simulink model "QPSK_ad9361_LNA"  (R2017b)
settings: Solver=ode23  StartTime=0.0  StopTime=inf  RelTol=1e-3  EnableMultiTasking=on
PreLoadFcn:
  | addpath('./filterwizard');
  | adi9361_preload(bdroot,'rx');
  | sdrqpsktx = sdrzqpsktxFMC234_init;
  | sdrqpskrx = sdrzqpskrxFMC234_init;
InitFcn:
  | sdrqpsktx = sdrzqpsktxFMC234_init;
  | sdrqpskrx = sdrzqpskrxFMC234_init;
undefined symbols (not defined in the file or in its folder): D, dBval, DCLeak_Matrix, dfilt, fuzz_val, GainImb_Matrix, gcbh, IP2_Matrix, IP3_Matrix, magnitude, rcfiltgaincompat
libraries: simrfV2elements x12, simulink x7, dsparch4 x6, dspmlti4 x5, simrfV2util1 x4, fl_lib x4, simrfV2junction1 x3, dspsrcs4 x3, dspmathops x3, commdigbbndpm3 x3, dspstat3 x3, dspobslib x3
(part 1 of 3)
settings Model: SimulationMode=accelerator  Creator=The MathWorks Inc.  LastModifiedBy=ppradhan
settings DataIOCC: ExternalInput=txWaveform  SaveFormat=StructureWithTime  SaveOutput=off  SignalLogging=off  DSMLogging=off  SaveTime=off  OutputSaveName=rx
settings OptimizationCC: DefaultParameterBehavior=Inlined  InlineInvariantSignals=on  EfficientMapNaN2IntZero=off  LifeSpan=inf  SimCompilerOptimization=on
settings DebuggingCC: ReadBeforeWriteMsg=DisableAll  WriteAfterWriteMsg=DisableAll  WriteAfterReadMsg=DisableAll  UnderspecifiedInitializationDetection=Classic  MergeDetectMultiDrivingBlocksExec=none  SolverPrmCheckMsg=warning  InheritedTsInSrcMsg=none  MultiTaskDSMMsg=none  IntegerOverflowMsg=none  AllowSymbolicDim=off  SFUnexpectedBacktrackingDiag=warning  SFNoUnconditionalDefaultTransitionDiag=none  SFUndirectedBroadcastEventsDiag=none  SFExecutionAtInitializationDiag=none  IntegerSaturationMsg=none
settings HardwareCC: ProdBitPerPointer=32  ProdBitPerSizeT=32  ProdBitPerPtrDiffT=32  ProdLargestAtomicFloat=None  ProdIntDivRoundTo=Undefined  ProdEndianess=Unspecified  ProdWordSize=32  ProdHWDeviceType=32-bit Generic  TargetBitPerPointer=64  TargetBitPerSizeT=64  TargetBitPerPtrDiffT=64  TargetLongLongMode=on  TargetIntDivRoundTo=Zero  TargetEndianess=LittleEndian  TargetWordSize=64  TargetHWDeviceType=MATLAB Host  ProdEqTarget=off
settings ModelReferenceCC: UpdateModelReferenceTargets=IfOutOfDate  PropagateSignalLabelsOutOfModel=off
settings SFSimCC: SFSimEcho=off
settings CodeAppCC: MaxIdLength=128  StateflowObjectComments=on
settings GRTTargetCC: TargetLangStandard=C89/C90 (ANSI)  GeneratePreprocessorConditionals=Disable all  CombineOutputUpdateFcns=off  GRTInterface=on
settings ConfigComp: CovMetricSettings=dw  CovHtmlReporting=on  CovSaveCumulativeToWorkspaceVar=on  CovSaveSingleToWorkspaceVar=on  CovExternalEMLEnable=off  CovSFcnEnable=off
settings SimscapeCC: ExplicitSolverDiagnosticOptions=none

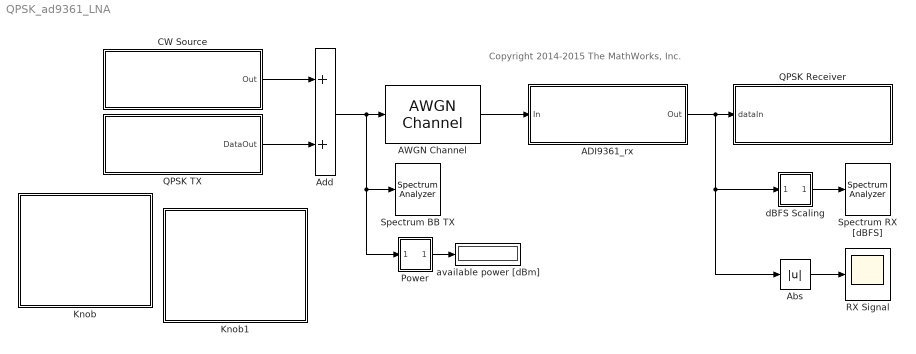
== system QPSK_ad9361_LNA ==
  note: Copyright 2014-2015 The MathWorks, Inc.
  ADI9361_rx : Subsystem  mask(ADI9361_RX){TestSignal=Custom, LOFreq=2e9, Ovs=2}
      mask prompts: TestSignal "Filter Configuration:"; LOFreq "LO Frequency (Hz):"; Ovs "Oversampling"
      mask help: Model an Analog Devices AD9361 RF Receiver.
      mask init:
      | ad9361_rx_pars = ad9361_rx_initfcn(gcb,'Init');
      | assignin('base', 'ad9361_rx_hm1Filt', ad9361_rx_pars.ad9361_rx_hm1Filt);
      | assignin('base', 'ad9361_rx_hm2Filt', ad9361_rx_pars.ad9361_rx_hm2Filt);
      | assignin('base', 'ad9361_rx_hm3Filt', ad9361_rx_pars.ad9361_rx_hm3Filt);
      | assignin('base', 'ad9361_rx_hm4Filt', ad9361_rx_pars.ad9361_rx_hm4Filt);
      | Trf = evalin('base','sdrqpskrx.RadioFrontEndSamplePeriod')/Ovs;
      | load ADI9361Tables;
      | iip3_800MHz  = [10, 10, 10, 8,   8,   10,  9,   -3, -5, -5, -8, -13, -14, -18];
      | iip3_2p4GHz  = [9,  9,   9,   8,   7,    9,   8,   0,   0,  -5, -5, -7,   -8,   -10];
      | iip3_5p5GHz  = [16,10, 10, 11,  11, 11, 11,  11, 11, -3, -6, -7,  -10, -16];
      | 
      | iip2_800MHz  = [80, 80, 80, 58, 48];
      | iip2_2p4GHz  = [70, 70, 70, 60, 50];
      | iip2_5p5GHz  = [70, 70, 70, 60, 45];
      | 
      | if LOFreq<=1.3e9
      |     IIP3 = iip3_800MHz;
      |     IIP2 = iip2_800MHz;
      | elseif LOFreq <= 4e9
      |     IIP3 = iip3_2p4GHz;
      |     IIP2 = iip2_2p4GHz;
      | else
      |     IIP3 = iip3_5p5GHz;
      |     IIP2 = iip2_5p5GHz;
      | end
      | IP3_Matrix(:,5)=IIP3(:);
      | IP2_Matrix(:,5)=IIP2(:);
      mask Help:
      | Model an Analog Devices AD9361 RF Receiver. This model predicts thermal noise, spectral growth, LO carrier leakage and image signals, quantization noise in manual and slow attack control mode.
      | 
      | To change the automatic gain control mode, toggle the manual switch between manual mode and slow-attack control mode under the receiver mask. For manual mode, directly specify the index of the gain table in the constant block "manual index".
      | 
      | For signals with LTE 5MHz, LTE 10 MHz and LTE 20 MHz characteristics, the default configurations recommended by Analog Devices are directly available.
      | 
      | The filters are programmable. Use the Analog Devices Wizard App to custom design Filters. Select the option “Custom” in the “ Filter Configuration” menu and click “Design Filter” button. The Filter Design app will open automatically. Make sure a receiver filter is designed instead of a transmitter filter. After designing the filter, click the button “Export to Workspace” in the App. The custom filter design is saved in the model set up. Next time a simulation is setup with custom filter configuration, the latest filter design is used.
      | 
      | Make sure that the input signal sample time and the expected step size of the RF simulation are the same. In case of a mismatch, an error is generated.
      mask TypeOptions TestSignal: 5MHz LTE | 10MHz LTE | 20MHz LTE | Custom
      mask Callback TestSignal:
      | % Set Mask visibilites and enables
      | ad9361_rx_mask_callbacks(gcb,'TestSignal')
      mask DialogControl Control2 Prompt: SpacerDesign
      mask DialogControl DesignFilter Prompt: Design Filter
      mask DialogControl DesignFilter Callback: ad9361_rx_initfcn(gcb,'DesignFilter');
      mask Display: text(0.5,0.5,'AD9361_RX','horizontalAlignment','center');
  AWGN Channel : commchan3/AWGN Channel  InputProcessing=Columns as channels (frame based)  seed=67  noiseMode="Signal to noise ratio  (SNR)"  EbNodB=10  EsNodB=10  SNRdB=3  bitsPerSym=1  Ps=1e-13*(50)  Tsym=1  variance=1
  Abs : Abs
  Add : Sum
  CW Source : Subsystem  mask{Sel=CW + 100kHz tone, CW=120e3, Power=-100, Ovs=2}
      mask prompts: Sel "Select source"; CW "Frequency (Hz)"; Power "Power (dBm)"; Ovs "Oversampling"
      mask init:
      | Tstep = evalin('base','sdrqpskrx.RadioFrontEndSamplePeriod');
      mask TypeOptions Sel: CW + 100kHz tone | Single CW tone | Dual CW tone
      mask DialogControl DescGroupVar Prompt: Ideal Test Source
      mask Display: disp('CW Source')
  Knob : Subsystem  DialogController=hmiCreateDDGDialog  IsWebBlock=on  mask(MathWorksWebBlock){webBlockId=10992aa7-3387-4369-8f6d-c1f2990169a8, webBlockType=continuousknob, ShowInLibBrowser=on, ShowInitialText=on, HMISrcModelName=QPSK_ad9361_LNA}
      mask prompts: webBlockId "WebBlock Id"; webBlockType "WebBlock Type"; HMISrcModelName "Source Model"
      mask Help: helpview([docroot '/mapfiles/simulink.map'], 'hmi_knob')
      mask Display:
      | if strcmp(get_param(bdroot(gcb),'BlockDiagramType'), 'library')
      |     image([(matlabroot) '/toolbox/simulink/hmi/icons/ContinuousKnob.png']);
      | end
  Knob1 : Subsystem  DialogController=hmiCreateDDGDialog  IsWebBlock=on  mask(MathWorksWebBlock){webBlockId=33e80c37-c5c4-41e7-8880-b6785ebea8d0, webBlockType=continuousknob, ShowInLibBrowser=on, ShowInitialText=on, HMISrcModelName=QPSK_ad9361_LNA}
      mask prompts: webBlockId "WebBlock Id"; webBlockType "WebBlock Type"; HMISrcModelName "Source Model"
      mask Help: helpview([docroot '/mapfiles/simulink.map'], 'hmi_knob')
      mask Display:
      | if strcmp(get_param(bdroot(gcb),'BlockDiagramType'), 'library')
      |     image([(matlabroot) '/toolbox/simulink/hmi/icons/ContinuousKnob.png']);
      | end
  "Power  " : Subsystem  mask{R=50}
      mask prompts: R "Reference Impedance [Ohm]"
      mask DialogControl DescGroupVar Prompt: Power Meter
  QPSK Receiver : Subsystem
      mask Display: disp('QPSK Receiver');
  QPSK TX : Subsystem  mask{Ovs=2, Power=-100}
      mask prompts: Ovs "Oversampling"; Power "Power (dBm)"
      mask Display: disp('QPSK Transmitter')
  RX Signal : Scope
  Spectrum BB TX : SpectrumAnalyzer
  Spectrum RX [dBFS] : SpectrumAnalyzer
  available power [dBm] : Display
  dBFS Scaling : Subsystem
  wires:
  CW Source/1(Out) -> Add/1
  "Power  "/1(Out) -> available power [dBm]/1
  dBFS Scaling/1(Out) -> Spectrum RX [dBFS]/1
  Abs/1 -> RX Signal/1
  ADI9361_rx/1(Out) -> QPSK Receiver/1(dataIn), dBFS Scaling/1(In), Abs/1
  Add/1 -> AWGN Channel/1, Spectrum BB TX/1, "Power  "/1(In)
  QPSK TX/1(DataOut) -> Add/2
  AWGN Channel/1 -> ADI9361_rx/1(In)

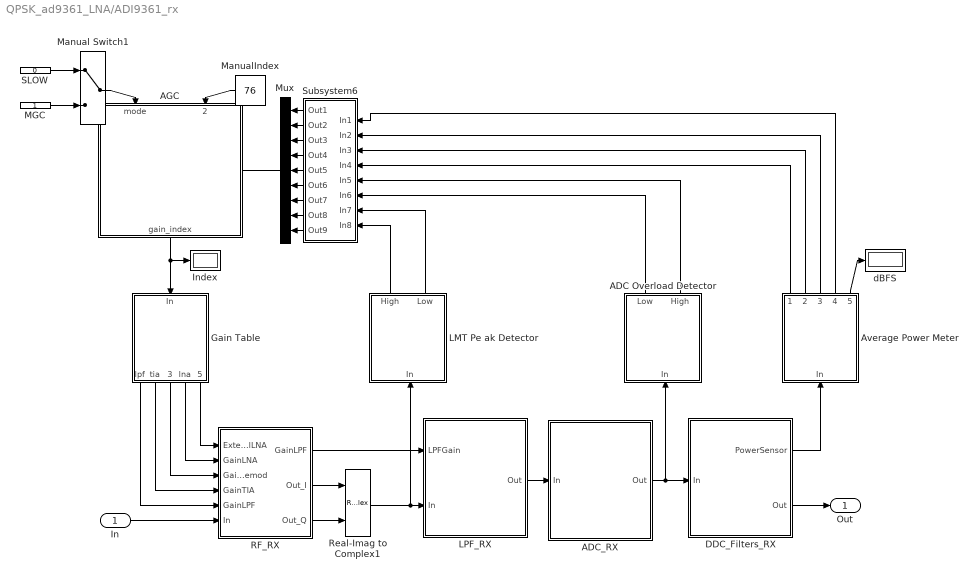
== system QPSK_ad9361_LNA/ADI9361_rx ==
  In : Inport
  ADC Overload Detector : Subsystem  mask{Ncycles=4, Lthreshold=47, Hthreshold=58}
      mask prompts: Ncycles "Number of Integration Cycles"; Lthreshold "Low Threshold"; Hthreshold "High Threshold"
      mask DialogControl DescGroupVar Prompt: ADC Overload Detector
  ADC_RX : Subsystem
  AGC : Stateflow chart  TreatAsAtomicUnit=on  mask{N_LMT_H=10, N_LMT_L=10, LMT_G_dec_fast=2, N_ADC_H=10, N_ADC_L=10, ADC_G_dec_fast=2, AGC_G_inc_fast=2, AGC_G_inc_slow=1, AGC_G_dec_fast=2, AGC_G_dec_slow=1, C=100, T=1}
      mask prompts: N_LMT_H "LMT Upper Count"; N_LMT_L "LMT Lower Count"; LMT_G_dec_fast "LMT Gain index decrement - outer"; N_ADC_H "ADC Upper Count"; N_ADC_L "ADC Lower Count"; ADC_G_dec_fast "ADC - Gain index decrement - outer"; AGC_G_inc_fast "AGC - Gain index increment - outer"; AGC_G_inc_slow "AGC - Gain index increment - inner"; AGC_G_dec_fast "AGC - Gain index decrement - outer"; AGC_G_dec_slow "AGC - Gain index decrement - inner"; C "Gain Update Interval for Slow Mode [us]"; T "Extra delay margin [us]"
  Average Power Meter : Subsystem  mask{Ncycles=1024 %8192, Hthreshold_o=-5, Hthreshold_i=-10, Lthreshold_i=-12, Lthreshold_o=-18}
      mask prompts: Ncycles "Number of Integration Cycles"; Hthreshold_o "Outer High Threshold [dBFS]"; Hthreshold_i "Inner High Threshold [dBFS]"; Lthreshold_i "Inner Low Threshold [dBFS]"; Lthreshold_o "Outer Low Threshold [dBFS]"
      mask DialogControl DescGroupVar Prompt: AGC Low Power Detector
  DDC_Filters_RX : Subsystem
  Gain Table : Subsystem
  "Index " : Display
  LMT Pe ak Detector : Subsystem  mask{HThreshold=800, LThreshold=704}
      mask prompts: HThreshold "High Threshold [mV]"; LThreshold "Low Threshold [mV]"
      mask DialogControl DescGroupVar Prompt: LMT Peak Detector
  LPF_RX : Subsystem
  MGC : Constant  SampleTime=-1
  Manual Switch1 : ManualSwitch
  ManualIndex : Constant  Value=76  SampleTime=-1
  Mux : Mux  Inputs=9
  RF_RX : Subsystem  mask{RF=LOFreq, Tstep=Trf}
      mask prompts: RF "Center Frequency [Hz]"; Tstep "Sample Time [s]"
      mask init:
      | freq = [0.8e9, 2.4e9, 5.5e9];
      | nf   = [2,       3,        3.8];
      | NF   = interp1(freq, nf, RF,'linear','extrap');
      | 
      | S11 = -200;
      | Rin = s2z(10^(S11/20));
      mask DialogControl DescGroupVar Prompt: ADI 9361 Receiver RF Parameters
  Real-Imag to Complex1 : RealImagToComplex
  SLOW : Constant  Value=0  SampleTime=-1
  Subsystem6 : Subsystem
  dBFS : Display
  Out : Outport
  wires:
  RF_RX/2(Out_I) -> Real-Imag to Complex1/1
  RF_RX/3(Out_Q) -> Real-Imag to Complex1/2
  Real-Imag to Complex1/1 -> LMT Pe ak Detector/1(In), LPF_RX/2(In)
  Gain Table/2(tia) -> RF_RX/4(GainTIA)
  Gain Table/3(demod) -> RF_RX/3(GainDemod)
  Gain Table/4(lna) -> RF_RX/2(GainLNA)
  LPF_RX/1(Out) -> ADC_RX/1(In)
  MGC/1 -> Manual Switch1/2
  SLOW/1 -> Manual Switch1/1
  Manual Switch1/1 -> AGC/1(mode)
  LMT Pe ak Detector/2(Low) -> Subsystem6/7(In7)
  Gain Table/1(lpf) -> RF_RX/5(GainLPF)
  DDC_Filters_RX/1(PowerSensor) -> Average Power Meter/1(In)
  ADC Overload Detector/2(High) -> Subsystem6/5(In5)
  Average Power Meter/1(Outer_High) -> Subsystem6/4(In4)
  Average Power Meter/2(Inner_High) -> Subsystem6/3(In3)
  Average Power Meter/3(Inner_Low) -> Subsystem6/2(In2)
  Average Power Meter/4(Outer_Low) -> Subsystem6/1(In1)
  LMT Pe ak Detector/1(High) -> Subsystem6/8(In8)
  Subsystem6/1(Out1) -> Mux/1
  Subsystem6/2(Out2) -> Mux/2
  Subsystem6/3(Out3) -> Mux/3
  Subsystem6/4(Out4) -> Mux/4
  Subsystem6/5(Out5) -> Mux/5
  Subsystem6/8("Out8 ") -> Mux/8
  ADC Overload Detector/1(Low) -> Subsystem6/6(In6)
  Subsystem6/6(Out6) -> Mux/6
  Subsystem6/7(Out7) -> Mux/7
  DDC_Filters_RX/2(Out) -> Out/1
  Average Power Meter/5(Power [dBFS]) -> dBFS/1
  Subsystem6/9(Out9) -> Mux/9
  In/1 -> RF_RX/6(In)
  AGC/1(gain_index) -> "Index "/1, Gain Table/1(In)
  ManualIndex/1 -> AGC/2(ManualGainIndex)
  Mux/1 -> AGC/Trigger
  RF_RX/1("GainLPF ") -> LPF_RX/1(LPFGain)
  Gain Table/5(External LNA) -> RF_RX/1(ExternalLNA)
  ADC_RX/1(Out) -> ADC Overload Detector/1(In), DDC_Filters_RX/1(In)

== system QPSK_ad9361_LNA/CW Source ==
  2Tones : dspsrcs4/Sine Wave  Amplitude=sqrt(2)  Frequency=CW/2  Phase=0  SampleMode=Discrete  OutComplex=Real  CompMethod=Trigonometric fcn  TableSize=Speed  SampleTime=Tstep/Ovs  SamplesPerFrame=1  ResetState=Restart at time zero  OutputFrames=on  dataType=double  wordLen=16  udDataType=sfix(16)  fracBitsMode=Best precision  numFracBits=15  OutDataTypeStr=double  LastOutDataTypeStr=double
  CW : dspsrcs4/Sine Wave  Amplitude=1  Frequency=CW  Phase=0  SampleMode=Discrete  OutComplex=Complex  CompMethod=Trigonometric fcn  TableSize=Speed  SampleTime=Tstep/Ovs  SamplesPerFrame=1  ResetState=Restart at time zero  OutputFrames=on  dataType=double  wordLen=16  udDataType=sfix(16)  fracBitsMode=Best precision  numFracBits=15  OutDataTypeStr=double  LastOutDataTypeStr=double
  CW+Modulation : dspsrcs4/Sine Wave  Amplitude=[1; 1]/sqrt(2)  Frequency=[CW; 100e3]  Phase=[0; 0]  SampleMode=Discrete  OutComplex=Complex  CompMethod=Trigonometric fcn  TableSize=Speed  SampleTime=Tstep/Ovs  SamplesPerFrame=1  ResetState=Restart at time zero  OutputFrames=on  dataType=double  wordLen=16  udDataType=sfix(16)  fracBitsMode=Best precision  numFracBits=15  OutDataTypeStr=double  LastOutDataTypeStr=double
  Constant : Constant  Value=Sel  SampleTime=Tstep/Ovs
  Multiport Switch : MultiPortSwitch
  Real-Imag to Complex : RealImagToComplex  Input=Real
  Sum of Elements : Sum  Inputs=+
  dB Gain : dspmathops/dB Gain  dB=Power-30+20*log10(sqrt(50))  intype=Amplitude
      settings: SourceProductName=DSP System Toolbox  SourceProductBaseCode=DS
  Out : Outport
  wires:
  dB Gain/1 -> Out/1
  Multiport Switch/1 -> dB Gain/1
  Real-Imag to Complex/1 -> Multiport Switch/4
  Constant/1 -> Multiport Switch/1
  2Tones/1 -> Real-Imag to Complex/1
  CW/1 -> Multiport Switch/3
  Sum of Elements/1 -> Multiport Switch/2
  CW+Modulation/1 -> Sum of Elements/1

== system QPSK_ad9361_LNA/Knob ==

== system QPSK_ad9361_LNA/Knob1 ==

== system QPSK_ad9361_LNA/Power   ==
  In : Inport
  CountNCycles : Buffer  N=1024
  Frame Conversion : FrameConversion  InheritSamplingMode=off  OutFrame=Sample-based
  Gain2 : Gain  Gain=1/1024
  Root : Sqrt  SaturateOnIntegerOverflow=on
  Squared : Math  Operator=magnitude^2  SaturateOnIntegerOverflow=on
  Sum : Sum  Inputs=+
  dB Conversion : dspmathops/dB Conversion  dBtype=dBm  intype=Amplitude  R=R  fuzz=on
      settings: SourceProductName=DSP System Toolbox
  Out : Outport
  wires:
  dB Conversion/1 -> Out/1
  In/1 -> CountNCycles/1
  Frame Conversion/1 -> dB Conversion/1
  CountNCycles/1 -> Squared/1
  Squared/1 -> Sum/1
  Sum/1 -> Gain2/1
  Root/1 -> Frame Conversion/1
  Gain2/1 -> Root/1

== system QPSK_ad9361_LNA/QPSK Receiver ==
  note: Receiver
  dataIn : Inport
  Coarse Frequency Compensation : Subsystem
      mask Display: disp('Coarse Frequency\nCompensation');
  Data Decoding : Subsystem
      mask Display: disp('Data Decoding');
  Fine Frequency Compensation : Subsystem
      mask Display: disp('Fine Frequency\nCompensation')
  Gain : Gain  Gain=4/2047*sqrt(sdrqpskrx.Upsampling)/sqrt(2)
  Raised Cosine Receive Filter : commfilt2/Raised Cosine Receive Filter  filtType=Square root  R=0.5  filtSpan=2*((sdrqpskrx.RCFiltSpan)/2)  N=sdrqpskrx.Upsampling  downFactor=sdrqpskrx.Downsampling  downOffset=0  filterGain=rcfiltgaincompat(gcbh)  RateOptions=Allow multirate processing  framing=Mute  checkCoeff=off  variableName=rcRxFilt1  currentFiltSpan=2*((sdrqpskrx.RCFiltSpan)/2)  D=(sdrqpskrx.RCFiltSpan)/2  inputOffset=0  sampMode=Mute  saveAsFlag=0  rateMode=Downsampling  checkGain=Normalized  launchFVT=off  roundingMode=Floor  overflowMode=off  coeffDataTypeStr=Inherit: Same word length as input  coeffMin=[]  coeffMax=[]  coeffLastDataTypeStr=Inherit: Same word length as input  accumDataTypeStr=Inherit: Same as product output  accumLastDataTypeStr=Inherit: Same as product output  outputDataTypeStr=Inherit: Same as accumulator  outputMin=[]  outputMax=[]  outputLastDataTypeStr=Inherit: Same as accumulator
  Timing Recovery : Subsystem
      mask Display:
      | disp('Timing\nRecovery');
      | port_label('output',1,'DataOut');
      | port_label('output',2,'DataValid');
  Zero-Order Hold : ZeroOrderHold  SampleTime=sdrqpskrx.RadioFrontEndSamplePeriod
  wires:
  Timing Recovery/1(Out) -> Data Decoding/1(In)
  Timing Recovery/2(DataValid) -> Data Decoding/Trigger
  Raised Cosine Receive Filter/1 -> Coarse Frequency Compensation/1(In)
  Coarse Frequency Compensation/1(Out) -> Fine Frequency Compensation/1(In)
  Fine Frequency Compensation/1(Out) -> Timing Recovery/1(In)
  dataIn/1 -> Zero-Order Hold/1
  Gain/1 -> Raised Cosine Receive Filter/1
  Zero-Order Hold/1 -> Gain/1

== system QPSK_ad9361_LNA/QPSK TX ==
  note: Upsample by 4
  Bit Generation : Subsystem
      mask Display: disp('Bits Generation')
  "Interpolation " : Subsystem
  QPSK Modulator Baseband : commdigbbndpm3/QPSK Modulator Baseband  InType=Bit  Enc=Gray  Ph=pi/4  outDtype=double  outWordLen=16  outUDDataType=sfix(16)  outFracLenMode=Best precision  outFracLen=15
  Raised Cosine Transmit Filter : commfilt2/Raised Cosine Transmit Filter  filtType=Square root  R=0.5  filtSpan=2*((sdrqpsktx.RCFiltSpan)/2)  N=sdrqpsktx.Upsampling  filterGain=rcfiltgaincompat(gcbh)  InputProcessing=Columns as channels (frame based)  RateOptions=Enforce single-rate processing  framing=Mute  checkCoeff=off  variableName=rcTxFilt1  checkGain=Normalized  sampMode=Mute  saveAsFlag=0  currentFiltSpan=2*((sdrqpsktx.RCFiltSpan)/2)  D=(sdrqpsktx.RCFiltSpan)/2  launchFVT=off  roundingMode=Floor  overflowMode=off  coeffDataTypeStr=Inherit: Same word length as input  coeffMin=[]  coeffMax=[]  coeffLastDataTypeStr=Inherit: Same word length as input  outputDataTypeStr=Inherit: Same as accumulator  outputMin=[]  outputMax=[]  outputLastDataTypeStr=Inherit: Same as accumulator
  Unbuffer : Unbuffer
  dB Gain : dspmathops/dB Gain  dB=Power-30+20*log10(sqrt(50))+6+0.17  intype=Amplitude
      settings: SourceProductName=DSP System Toolbox  SourceProductBaseCode=DS
  DataOut : Outport
  wires:
  Unbuffer/1 -> "Interpolation "/1(In)
  QPSK Modulator Baseband/1 -> Raised Cosine Transmit Filter/1
  Raised Cosine Transmit Filter/1 -> dB Gain/1
  Bit Generation/1(Out) -> QPSK Modulator Baseband/1
  dB Gain/1 -> Unbuffer/1
  "Interpolation "/1(Out) -> DataOut/1

== system QPSK_ad9361_LNA/dBFS Scaling ==
  In : Inport
  Gain : Gain  Gain=1/2047
  Out : Outport
  wires:
  In/1 -> Gain/1
  Gain/1 -> Out/1

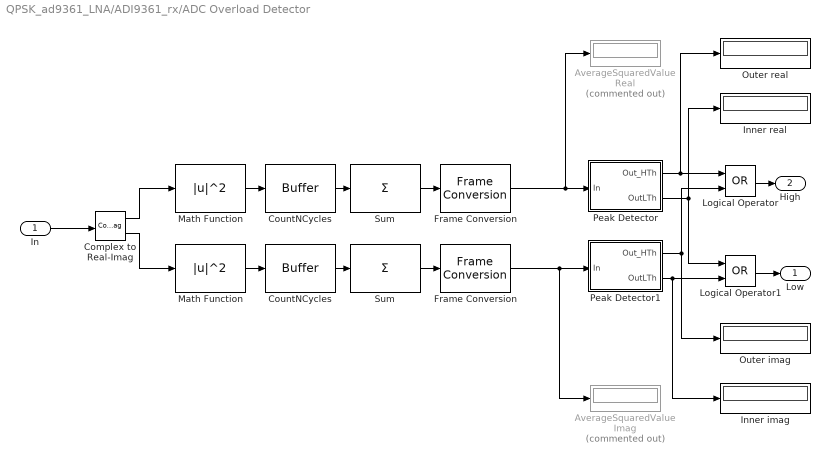
== system QPSK_ad9361_LNA/ADI9361_rx/ADC Overload Detector ==
  In : Inport
  AverageSquaredValue Imag : Display  Commented=on
  AverageSquaredValue Real : Display  Commented=on
  Complex to Real-Imag : ComplexToRealImag
  CountNCycles : Buffer  N=Ncycles
  "CountNCycles " : Buffer  N=Ncycles
  Frame Conversion : FrameConversion  InheritSamplingMode=off  OutFrame=Sample-based
  "Frame Conversion " : FrameConversion  InheritSamplingMode=off  OutFrame=Sample-based
  Inner imag : Display
  Inner real : Display
  Logical Operator : Logic  Operator=OR  AllPortsSameDT=off  OutDataTypeStr=boolean
  Logical Operator1 : Logic  Operator=OR  AllPortsSameDT=off  OutDataTypeStr=boolean
  Math Function : Math  Operator=magnitude^2  SaturateOnIntegerOverflow=on
  "Math Function " : Math  Operator=magnitude^2  SaturateOnIntegerOverflow=on
  Outer imag : Display
  Outer real : Display
  Peak Detector : Subsystem  mask{HThreshold=Hthreshold, LThreshold=Lthreshold}
      mask prompts: HThreshold "High Threshold (bit string) <4:0>"; LThreshold "Low Threshold (bit string) <4:0>"
  Peak Detector1 : Subsystem  mask{HThreshold=Hthreshold, LThreshold=Lthreshold}
      mask prompts: HThreshold "High Threshold (bit string) <4:0>"; LThreshold "Low Threshold (bit string) <4:0>"
  Sum : Sum  Inputs=+
  "Sum " : Sum  Inputs=+
  Low : Outport
  High : Outport  Port=2
  wires:
  Math Function/1 -> CountNCycles/1
  CountNCycles/1 -> Sum/1
  Sum/1 -> Frame Conversion/1
  Frame Conversion/1 -> AverageSquaredValue Real/1, Peak Detector/1(In)
  In/1 -> Complex to Real-Imag/1
  "Math Function "/1 -> "CountNCycles "/1
  "CountNCycles "/1 -> "Sum "/1
  "Sum "/1 -> "Frame Conversion "/1
  "Frame Conversion "/1 -> AverageSquaredValue Imag/1, Peak Detector1/1(In)
  Peak Detector/2(OutLTh) -> Logical Operator1/1, Inner real/1
  Peak Detector/1(Out_HTh) -> Outer real/1, Logical Operator/1
  Peak Detector1/1(Out_HTh) -> Logical Operator/2, Outer imag/1
  Peak Detector1/2(OutLTh) -> Inner imag/1, Logical Operator1/2
  Logical Operator/1 -> High/1
  Logical Operator1/1 -> Low/1
  Complex to Real-Imag/1 -> Math Function/1
  Complex to Real-Imag/2 -> "Math Function "/1

== system QPSK_ad9361_LNA/ADI9361_rx/ADC_RX ==
  In : Inport
  ADC_I : Subsystem
  ADC_Q : Subsystem
  Complex to Real-Imag1 : ComplexToRealImag
  Real-Imag to Complex : RealImagToComplex
  Out : Outport
  wires:
  Complex to Real-Imag1/1 -> ADC_I/1(In)
  Complex to Real-Imag1/2 -> ADC_Q/1(In)
  In/1 -> Complex to Real-Imag1/1
  Real-Imag to Complex/1 -> Out/1
  ADC_I/1(Out) -> Real-Imag to Complex/1
  ADC_Q/1(Out) -> Real-Imag to Complex/2

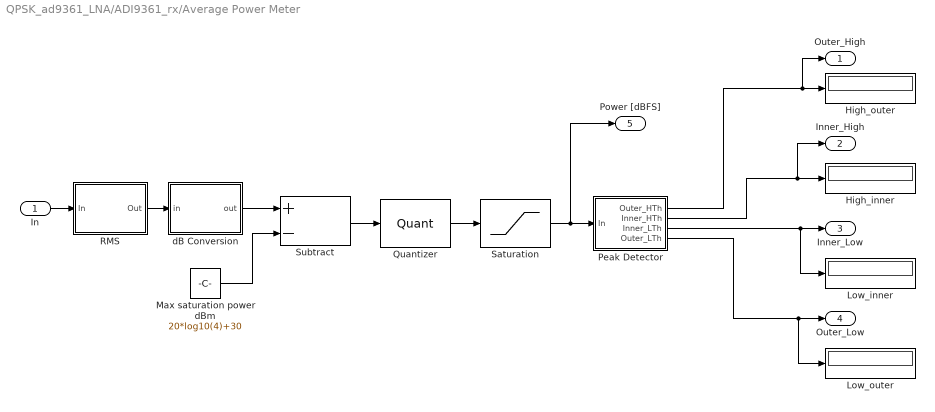
== system QPSK_ad9361_LNA/ADI9361_rx/Average Power Meter ==
  In : Inport
  High_inner : Display
  High_outer : Display
  Low_inner : Display
  Low_outer : Display
  Max saturation power dBm : Constant  Value=20*log10(4)+30  SampleTime=ad9361_rx_pars.Tpow*Ncycles
  Peak Detector : Subsystem  mask{HThreshold_o=Hthreshold_o, HThreshold_i=Hthreshold_i, LThreshold_i=Lthreshold_i, LThreshold_o=Lthreshold_o}
      mask prompts: HThreshold_o "Outer High Threshold (bit string) <4:0>"; HThreshold_i "Inner High Threshold (bit string) <4:0>"; LThreshold_i "Inner Low Threshold (bit string) <4:0>"; LThreshold_o "Outer Low Threshold (bit string) <4:0>"
  Quantizer : Quantizer
  RMS : Subsystem
  Saturation : Saturate  UpperLimit=0  LowerLimit=-63.5
  Subtract : Sum  Inputs=+-
  dB Conversion : Subsystem  mask(dB Conversion){dBtype=dBm, intype=Amplitude, R=1, fuzz=on}
      mask prompts: dBtype "Convert to:"; intype "Input signal:"; R "Load resistance (ohms):"; fuzz "Add eps to input to protect against  "log(0) = -inf""
      mask help: Convert input of watts or volts to decibels. Voltage inputs are first converted to power relative to the specified load resistance, where P = (V^2)/R. When converting to dB, the reference power is 1 W. When converting to dBm, the reference power is 1 mW.
      mask init:
      | [str fuzz_val dBval] = dspblkdb2('init');
      | dspblkdb2('checkparam');
      | dspblkdb2('update');
      mask Help: eval('blocksethelp');
      mask TypeOptions dBtype: dB | dBm
      mask Callback dBtype: dspblkdb2
      mask TypeOptions intype: Power | Amplitude
      mask Callback intype: dspblkdb2
      mask Display: disp(str)
  Outer_High : Outport  SampleTime=ad9361_rx_pars.Tpow*Ncycles
  Inner_High : Outport  Port=2  SampleTime=ad9361_rx_pars.Tpow*Ncycles
  Inner_Low : Outport  Port=3  SampleTime=ad9361_rx_pars.Tpow*Ncycles
  Outer_Low : Outport  Port=4  SampleTime=ad9361_rx_pars.Tpow*Ncycles
  Power [dBFS] : Outport  Port=5  SampleTime=ad9361_rx_pars.Tpow*Ncycles
  wires:
  Max saturation power dBm/1 -> Subtract/2
  Subtract/1 -> Quantizer/1
  Quantizer/1 -> Saturation/1
  Saturation/1 -> Power [dBFS]/1, Peak Detector/1(In)
  dB Conversion/1(out) -> Subtract/1
  Peak Detector/1(Outer_HTh) -> Outer_High/1, High_outer/1
  Peak Detector/2(Inner_HTh) -> Inner_High/1, High_inner/1
  Peak Detector/3(Inner_LTh) -> Inner_Low/1, Low_inner/1
  Peak Detector/4(Outer_LTh) -> Low_outer/1, Outer_Low/1
  In/1 -> RMS/1(In)
  RMS/1(Out) -> dB Conversion/1(in)

== system QPSK_ad9361_LNA/ADI9361_rx/DDC_Filters_RX ==
  In : Inport
  Data Type Conversion1 : DataTypeConversion  OutDataTypeStr=double
  Data Type Conversion2 : DataTypeConversion  OutDataTypeStr=double
  FIR Decimation : dspmlti4/FIR Decimation  FilterSource=Filter object  h=fir1(35,0.4)  D=2  filtStruct=Direct form  FilterObject=ad9361_rx_pars.Hmd_rx  framing=Allow multirate processing  inputOffset=0  outputBufInitCond=0  roundingMode=Floor  overflowMode=off  firstCoeffDataTypeStr=Inherit: Same word length as input  firstCoeffMin=[]  firstCoeffMax=[]  firstCoeffLastDataTypeStr=Inherit: Same word length as input  outputDataTypeStr=Inherit: Same as accumulator  outputMin=[]  outputMax=[]  outputLastDataTypeStr=Inherit: Same as accumulator
  Gain : Gain  Gain=1/4
  Gain1 : Gain  Gain=4
  Gain3 : Gain  Gain=2047/4
  Hm1 : Subsystem  Variant=on
  Hm2 : Subsystem  Variant=on
  Hm3 : Subsystem  Variant=on
  Hm4 : Subsystem  Variant=on
  PowerSensor : Outport
  Out : Outport  Port=2
  wires:
  In/1 -> Gain/1
  Hm4/1(Out1) -> Hm3/1(In)
  Hm3/1(Out) -> Hm2/1(In)
  Hm2/1(Out) -> Hm1/1(In)
  Hm1/1(Out) -> Data Type Conversion1/1, FIR Decimation/1
  FIR Decimation/1 -> Data Type Conversion2/1
  Gain3/1 -> Out/1
  Gain/1 -> Hm4/1(In1)
  Data Type Conversion1/1 -> Gain1/1
  Gain1/1 -> PowerSensor/1
  Data Type Conversion2/1 -> Gain3/1

== system QPSK_ad9361_LNA/ADI9361_rx/Gain Table ==
  In : Inport
  Delay1 : Delay  DelayLength=1  InitialCondition=76  SampleTime=Trf
  Demux : Demux  Outputs=6
  Direct Lookup Table (n-D) : LookupNDDirect  InputsSelectThisObjectFromTable=Column  Table=ADIGainTable'
  Index : Terminator
  lpf : Outport
  tia : Outport  Port=2
  demod : Outport  Port=3
  lna : Outport  Port=4
  External LNA : Outport  Port=5
  wires:
  Demux/3 -> demod/1
  Demux/2 -> lna/1
  Demux/4 -> tia/1
  Demux/5 -> lpf/1
  In/1 -> Delay1/1
  Delay1/1 -> Direct Lookup Table (n-D)/1
  Direct Lookup Table (n-D)/1 -> Demux/1
  Demux/6 -> External LNA/1
  Demux/1 -> Index/1

== system QPSK_ad9361_LNA/ADI9361_rx/LMT Pe ak Detector ==
  In : Inport
  Abs : Abs
  HTh : Constant  Value=HThreshold*1e-3
  "High " : Display
  HighThreshold : RelationalOperator  OutDataTypeStr=boolean  RndMeth=Nearest
  LTh : Constant  Value=LThreshold*1e-3
  Logical Operator : Logic  AllPortsSameDT=off  OutDataTypeStr=boolean
  Logical Operator1 : Logic  AllPortsSameDT=off  OutDataTypeStr=boolean
  "Low " : Display
  LowThreshold : RelationalOperator  OutDataTypeStr=boolean  RndMeth=Nearest
  Pulse Generator2 : DiscretePulseGenerator  SampleTime=Trf
  High : Outport  SampleTime=Trf
  Low : Outport  Port=2  SampleTime=Trf
  wires:
  LTh/1 -> LowThreshold/2
  Abs/1 -> HighThreshold/1, LowThreshold/1
  HTh/1 -> HighThreshold/2
  In/1 -> Abs/1
  HighThreshold/1 -> Logical Operator1/1, "High "/1
  LowThreshold/1 -> Logical Operator/2, "Low "/1
  Pulse Generator2/1 -> Logical Operator1/2, Logical Operator/1
  Logical Operator1/1 -> High/1
  Logical Operator/1 -> Low/1

== system QPSK_ad9361_LNA/ADI9361_rx/LPF_RX ==
  LPFGain : Inport
  In : Inport  Port=2
  AntiAliasing : dsparch4/Analog Filter Design  method=Butterworth  filttype=Lowpass  N=3  Wlo=1.4*ad9361_rx_pars.Fpass*2*pi  Whi=80  Rp=2  Rs=40
  "AntiAliasing " : dsparch4/Analog Filter Design  method=Butterworth  filttype=Lowpass  N=3  Wlo=1.4*ad9361_rx_pars.Fpass*2*pi  Whi=80  Rp=2  Rs=40
  Complex to Real-Imag : ComplexToRealImag
  Gain : Product
  Real-Imag to Complex1 : RealImagToComplex
  dB2lin : Subsystem
  Out : Outport
  wires:
  Complex to Real-Imag/1 -> AntiAliasing/1
  Real-Imag to Complex1/1 -> Out/1
  In/1 -> Gain/2
  LPFGain/1 -> dB2lin/1(In)
  Gain/1 -> Complex to Real-Imag/1
  dB2lin/1(Out) -> Gain/1
  "AntiAliasing "/1 -> Real-Imag to Complex1/2
  AntiAliasing/1 -> Real-Imag to Complex1/1
  Complex to Real-Imag/2 -> "AntiAliasing "/1

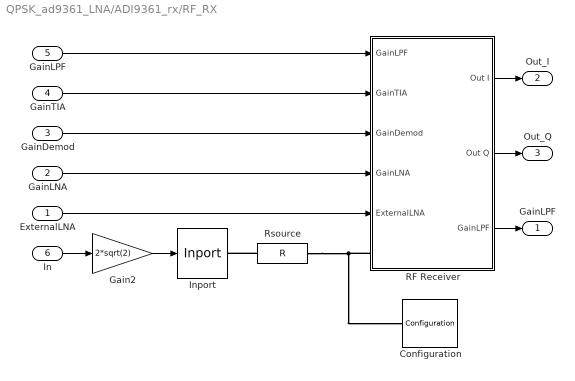
== system QPSK_ad9361_LNA/ADI9361_rx/RF_RX ==
  ExternalLNA : Inport
  GainLNA : Inport  Port=2
  GainDemod : Inport  Port=3
  GainTIA : Inport  Port=4
  GainLPF : Inport  Port=5
  In : Inport  Port=6
  Configuration : simrfV2util1/Configuration  AutoFreq=off  Tones=RF Hz  Harmonics=3  NormalizeCarrierPower=on  SolverType=Auto  StepSize=Tstep s  AddNoise=on  Temperature=290.0 K  SolverDelFlag=0
      settings: SourceProductName=RF Blockset  SourceProductBaseCode=RB
  Gain2 : Gain  Gain=2*sqrt(2)
  Inport : simrfV2util1/Inport  SimulinkInputSignalType=Ideal voltage  CarrierFreq=RF Hz  ZS=0  InternalGrounding=on
      settings: SourceProductName=RF Blockset  SourceProductBaseCode=RB
  RF Receiver : Subsystem
  Rsource : simrfV2elements/R  classname=resistor  Resistance=50 Ohm  AddNoise=on
      settings: SourceProductName=RF Blockset  SourceProductBaseCode=RB
  "GainLPF " : Outport
  Out_I : Outport  Port=2
  Out_Q : Outport  Port=3
  wires:
  In/1 -> Gain2/1
  GainTIA/1 -> RF Receiver/2(GainTIA)
  GainDemod/1 -> RF Receiver/3(GainDemod)
  GainLNA/1 -> RF Receiver/4(GainLNA)
  GainLPF/1 -> RF Receiver/1(GainLPF)
  Gain2/1 -> Inport/1
  RF Receiver/1(Out I) -> Out_I/1
  RF Receiver/2(Out Q) -> Out_Q/1
  RF Receiver/3("GainLPF ") -> "GainLPF "/1
  ExternalLNA/1 -> RF Receiver/5(ExternalLNA)
  connections:
  RF Receiver/LConn1 -- Rsource/LConn1 -- Configuration/LConn1
  Rsource/RConn1 -- Inport/RConn1

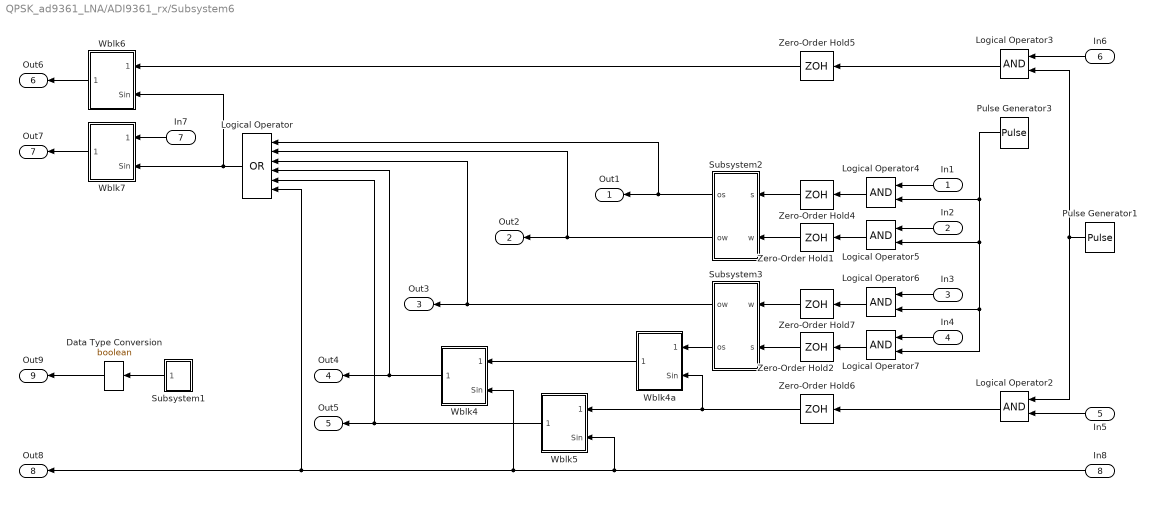
== system QPSK_ad9361_LNA/ADI9361_rx/Subsystem6 ==
  In1 : Inport
  In2 : Inport  Port=2
  In3 : Inport  Port=3
  In4 : Inport  Port=4
  In5 : Inport  Port=5
  In6 : Inport  Port=6
  In7 : Inport  Port=7
  In8 : Inport  Port=8
  Data Type Conversion : DataTypeConversion  OutDataTypeStr=boolean
  Logical Operator : Logic  Operator=OR  Inputs=6  AllPortsSameDT=off  OutDataTypeStr=boolean
  Logical Operator{2..6} (5 alike) : Logic  AllPortsSameDT=off  OutDataTypeStr=boolean
  Logical Operator7 : Logic  Priority=1  AllPortsSameDT=off  OutDataTypeStr=boolean
  Pulse Generator1 : DiscretePulseGenerator  SampleTime=ad9361_rx_pars.Tadc*4
  Pulse Generator3 : DiscretePulseGenerator  SampleTime=ad9361_rx_pars.Tpow*1024
  Subsystem1 : Subsystem
  Subsystem2 : Subsystem
  Subsystem3 : Subsystem
  Wblk4 : Subsystem
  Wblk4a : Subsystem
  Wblk5 : Subsystem
  Wblk6 : Subsystem
  Wblk7 : Subsystem
  Zero-Order Hold{1..2,4..7} (6 alike) : ZeroOrderHold  SampleTime=Trf
  Out1 : Outport
  Out2 : Outport  Port=2
  Out3 : Outport  Port=3
  Out4 : Outport  Port=4
  Out5 : Outport  Port=5
  Out6 : Outport  Port=6
  Out7 : Outport  Port=7
  "Out8 " : Outport  Port=8
  Out9 : Outport  Port=9
  wires:
  Subsystem3/2(os) -> Wblk4a/1(Win)
  Subsystem2/2(ow) -> Out2/1, Logical Operator/2
  Subsystem3/1(ow) -> Out3/1, Logical Operator/3
  Subsystem2/1(os) -> Out1/1, Logical Operator/1
  Wblk4a/1(Wout) -> Wblk4/1(Win)
  Logical Operator3/1 -> Zero-Order Hold5/1
  In7/1 -> Wblk7/1(Win)
  Logical Operator/1 -> Wblk7/2(Sin), Wblk6/2(Sin)
  Pulse Generator1/1 -> Logical Operator2/1, Logical Operator3/2
  Logical Operator2/1 -> Zero-Order Hold6/1
  Pulse Generator3/1 -> Logical Operator4/2, Logical Operator5/2, Logical Operator6/2, Logical Operator7/2
  Wblk7/1(Wout) -> Out7/1
  Wblk6/1(Wout) -> Out6/1
  Wblk4/1(Wout) -> Logical Operator/4, Out4/1
  Wblk5/1(Wout) -> Logical Operator/5, Out5/1
  Logical Operator4/1 -> Zero-Order Hold4/1
  Logical Operator6/1 -> Zero-Order Hold7/1
  Logical Operator5/1 -> Zero-Order Hold1/1
  Logical Operator7/1 -> Zero-Order Hold2/1
  Subsystem1/1(START) -> Data Type Conversion/1
  Data Type Conversion/1 -> Out9/1
  In1/1 -> Logical Operator4/1
  In2/1 -> Logical Operator5/1
  In3/1 -> Logical Operator6/1
  In4/1 -> Logical Operator7/1
  In5/1 -> Logical Operator2/2
  In6/1 -> Logical Operator3/1
  Zero-Order Hold5/1 -> Wblk6/1(Win)
  Zero-Order Hold4/1 -> Subsystem2/1(s)
  Zero-Order Hold1/1 -> Subsystem2/2(w)
  Zero-Order Hold7/1 -> Subsystem3/1(w)
  Zero-Order Hold2/1 -> Subsystem3/2(s)
  Zero-Order Hold6/1 -> Wblk4a/2(Sin), Wblk5/1(Win)
  In8/1 -> Wblk5/2(Sin), "Out8 "/1, Logical Operator/6, Wblk4/2(Sin)

== system QPSK_ad9361_LNA/QPSK Receiver/Coarse Frequency Compensation ==
  In : Inport
  Compensate for Frequency Offset : commrflib2/Phase// Frequency Offset  phaseOffset=0  freqPort=on  freqOffset=100
      settings: SourceProductName=Communications System Toolbox
  Find Frequency Offset : Subsystem  mask(Find Frequency Offset){M=sdrqpskrx.M, fftLen=2048, fftAvgs=16}
      mask prompts: M "Modulation order (integer):"; fftLen "FFT length (integer):"; fftAvgs "FFT averages (integer):"
  Out : Outport
  wires:
  In/1 -> Compensate for Frequency Offset/1, Find Frequency Offset/1(In)
  Compensate for Frequency Offset/1 -> Out/1
  Find Frequency Offset/1(Frq) -> Compensate for Frequency Offset/2

== system QPSK_ad9361_LNA/QPSK Receiver/Data Decoding ==
  note: Buffer one frame data in case that contiguous
      | data scatter across two adjacent frames
  note: This subsystem calculates the delay of the channel, align the data with
      | the detected frame head, resolves the possible phase ambiguity issue
      | during the fine frequency compensation and demodulates the data.
  note: Rx signal is delayed by (RxBufferedFrames+) frames.
      | The value 1 comes from one frame buffered at Data
      | Buffering subsystem with in the current subsystem
  In : Inport
  Trigger : TriggerPort  VariantControl=(inherit)  PortDimensions=1
  Align Data : MATLAB Function  TreatAsAtomicUnit=on
  "Barker Code Symbol Generation " : Subsystem
      mask Display: disp('Barker Code\nSymbol Generation')
  BitsToDecimal : MATLAB Function  TreatAsAtomicUnit=on
  Buffer : Buffer  N=sdrqpskrx.FrameSize*2  V=sdrqpskrx.FrameSize
  Compute Delay : Subsystem
      mask Display: disp('Compute\nDelay');
  Delay : Delay  DelayLength=1
  Delay1 : Delay  DelayLength=1
  Descrambling : Subsystem
      mask Display: disp('Descrambling')
  Phase Ambiguity Correction & Demodulation : Subsystem
      mask Display: disp('Phase Ambiguity\nCorrection\n& Demodulation');
  Phase Offset Estimator : Subsystem
  wires:
  Delay/1 -> Align Data/1(Delay)
  Buffer/1 -> Align Data/2(RxData)
  In/1 -> Compute Delay/2(Data), Buffer/1
  Compute Delay/1(Delay) -> Delay/1
  Align Data/1(Data) -> Phase Ambiguity Correction & Demodulation/2(Data), Phase Offset Estimator/2(Data)
  Phase Ambiguity Correction & Demodulation/1(Out) -> Descrambling/1(In)
  "Barker Code Symbol Generation "/1(Out) -> Compute Delay/1(Barker Reference), Phase Offset Estimator/1(BarkerRef)
  Phase Offset Estimator/1(Phase) -> Delay1/1
  Delay1/1 -> Phase Ambiguity Correction & Demodulation/1(Phase)
  Descrambling/1(Out) -> BitsToDecimal/1(u)

== system QPSK_ad9361_LNA/QPSK Receiver/Fine Frequency Compensation ==
  note: To determine the phase error detector gain K_p, See Equation 7.30 of "Digital
      | Communications - A Discrete-Time Approach" by Michael Rice.
  note: Baseband implementation of the QPSK Phase PLL listed in Figure 7.2.4 of
      | "Digital Communications - A Discrete-Time Approach" by Michael Rice. See
      | Appendix C.2 of the same book for the details of PLL design.
  In : Inport
  Complex Phase Shift : commutil2/Complex Phase Shift
      settings: SourceProductName=Communications System Toolbox  SourceProductBaseCode=CM
  DDS : Subsystem
      mask Display: disp('DDS')
  Delay1 : Delay  DelayLength=1  InitialCondition=0  InputProcessing=Columns as channels (frame based)
  Loop Filter : Subsystem  mask{BnTs=0.06, zeta=2.5, N=sdrqpskrx.Upsampling/sdrqpskrx.Downsampling, Kp=sdrqpskrx.FineFreqPEDGain, K0=sdrqpskrx.FineFreqCompensateGain}
      mask prompts: BnTs "Normalized Loop Bandwidth"; zeta "Damping Factor"; N "Number of Samples/Symbol"; Kp "Phase Detector Gain (Kp)"; K0 "DDS Gain (K0)"
      mask init:
      | % See C.57 to C.61 in Michael Rice's "Digital Communications 
      | % - A Discrete-Time Approach" for details
      | theta = BnTs/(zeta+0.25/zeta)/N;
      | d = 1 + 2*zeta*theta + theta*theta;
      | K1 = 4*zeta*theta/d;
      | K2 = 4*theta*theta/d;
      | K1 = K1/(Kp*K0);
      | K2 = K2/(Kp*K0);
      mask Display: disp('Loop Filter')
  PED : MATLAB Function  TreatAsAtomicUnit=on
  Unbuffer : Unbuffer
  Out : Outport
  wires:
  PED/1(e) -> Loop Filter/1(e)
  Loop Filter/1(v) -> DDS/1(In)
  DDS/1(Phase) -> Complex Phase Shift/2
  Unbuffer/1 -> Complex Phase Shift/1
  In/1 -> Unbuffer/1
  Complex Phase Shift/1 -> Delay1/1, Out/1
  Delay1/1 -> PED/1(In)

== system QPSK_ad9361_LNA/QPSK Receiver/Timing Recovery ==
  note: Baseband implementation of the Symbol Timing Synchronization listed in Chapter 8.4
      | of "Digital Communications- A Discrete-Time Approach" by Michael Rice. See
      | Appendix C.2 of the same book for the details of PLL design.
  note: MATLAB Implementation
      | of Scalar-based Timing Recovery
  In : Inport
  Modified Buffer : Subsystem  TreatAsAtomicUnit=on  mask(Input-Driven Buffer){bufSize=sdrqpskrx.FrameSize}
      mask prompts: bufSize "Buffer size:"
      mask help: A modified buffer subsystem that is driven by the arrival of its input data; it produces a valid output data buffer whenever its buffer is full and sets its dataValid flag to 1. Otherwise, the data at its dataOut port is not valid and its dataValid flag is set to 0.
  Timing Recovery PLL : Subsystem
      mask Display:
      | disp('Timing Recovery\nPLL')
      | port_label('input',1,'In')
      | port_label('output',1,'DataOut')
      | port_label('output',2,'Clk')
  Out : Outport
  DataValid : Outport  Port=2
  wires:
  Timing Recovery PLL/2(ClkOut) -> Modified Buffer/2(Clk)
  Timing Recovery PLL/1(DataOut) -> Modified Buffer/1(Data)
  In/1 -> Timing Recovery PLL/1(DataIn)
  Modified Buffer/1(DataOut) -> Out/1
  Modified Buffer/2(DataValid) -> DataValid/1

== system QPSK_ad9361_LNA/QPSK TX/Bit Generation ==
  note: Each data frame contains 26 bits header (For Sync Purpose) and 174 bits data bits,
      | first 105 bits contain "Hello world ###" message. Scrambler is there to improve data
      | transition density and frequency offset estimation.
  Barker Code SS : Subsystem
      mask Display: disp('Unipolar\nBarker Code')
  Matrix Concatenate : Concatenate  Mode=Multidimensional array
  Message Source : Subsystem
      mask Display: disp('Message\nSource')
  Repeat : dspsigops/Repeat  N=2  InputProcessing=Columns as channels (frame based)  RateOptions=Enforce single-rate processing  ic=0  mode=Unused parameter value
      settings: SourceProductName=DSP System Toolbox
  Scrambler : commsequence2/Scrambler  M=2  poly=[1 1 1 0 1]  iniStaSource=Dialog Parameter  ini_sta=[0 0 0 0]  resetViaPort=off
      settings: SourceProductName=Communications System Toolbox  SourceProductBaseCode=CM
  Out : Outport
  wires:
  Scrambler/1 -> Matrix Concatenate/2
  Repeat/1 -> Matrix Concatenate/1
  Message Source/1(Out) -> Scrambler/1
  Matrix Concatenate/1 -> Out/1
  Barker Code SS/1(Out) -> Repeat/1

== system QPSK_ad9361_LNA/QPSK TX/Interpolation  ==
  In : Inport
  AntiAliasing : dsparch4/Analog Filter Design  method=Elliptic  filttype=Lowpass  N=12  Wlo=2*pi/(4*sdrqpskrx.RadioFrontEndSamplePeriod)  Whi=80  Rp=0.1  Rs=120
  AntiAliasing1 : dsparch4/Analog Filter Design  method=Elliptic  filttype=Lowpass  N=12  Wlo=2*pi/(4*sdrqpskrx.RadioFrontEndSamplePeriod)  Whi=80  Rp=0.1  Rs=120
  Complex to Real-Imag : ComplexToRealImag
  Real-Imag to Complex1 : RealImagToComplex
  Zero-Order Hold1 : ZeroOrderHold  SampleTime=sdrqpskrx.RadioFrontEndSamplePeriod/Ovs
  Out : Outport
  wires:
  AntiAliasing1/1 -> Real-Imag to Complex1/2
  Complex to Real-Imag/2 -> AntiAliasing1/1
  Complex to Real-Imag/1 -> AntiAliasing/1
  In/1 -> Complex to Real-Imag/1
  AntiAliasing/1 -> Real-Imag to Complex1/1
  Real-Imag to Complex1/1 -> Zero-Order Hold1/1
  Zero-Order Hold1/1 -> Out/1

== system QPSK_ad9361_LNA/ADI9361_rx/ADC Overload Detector/Peak Detector ==
  In : Inport
  HTh : Constant  Value=Hthreshold  SampleTime=ad9361_rx_pars.Tadc*Ncycles
  HighThreshold : RelationalOperator  OutDataTypeStr=boolean  RndMeth=Nearest
  LTh : Constant  Value=Lthreshold  SampleTime=ad9361_rx_pars.Tadc*Ncycles
  LowThreshold : RelationalOperator  OutDataTypeStr=boolean  RndMeth=Nearest
  Out_HTh : Outport
  OutLTh : Outport  Port=2
  wires:
  LowThreshold/1 -> OutLTh/1
  HighThreshold/1 -> Out_HTh/1
  LTh/1 -> LowThreshold/2
  In/1 -> HighThreshold/1, LowThreshold/1
  HTh/1 -> HighThreshold/2

== system QPSK_ad9361_LNA/ADI9361_rx/ADC Overload Detector/Peak Detector1 ==
  In : Inport
  HTh : Constant  Value=Hthreshold  SampleTime=ad9361_rx_pars.Tadc*Ncycles
  HighThreshold : RelationalOperator  OutDataTypeStr=boolean  RndMeth=Nearest
  LTh : Constant  Value=Lthreshold  SampleTime=ad9361_rx_pars.Tadc*Ncycles
  LowThreshold : RelationalOperator  OutDataTypeStr=boolean  RndMeth=Nearest
  Out_HTh : Outport
  OutLTh : Outport  Port=2
  wires:
  HTh/1 -> HighThreshold/2
  In/1 -> LowThreshold/1, HighThreshold/1
  LTh/1 -> LowThreshold/2
  HighThreshold/1 -> Out_HTh/1
  LowThreshold/1 -> OutLTh/1

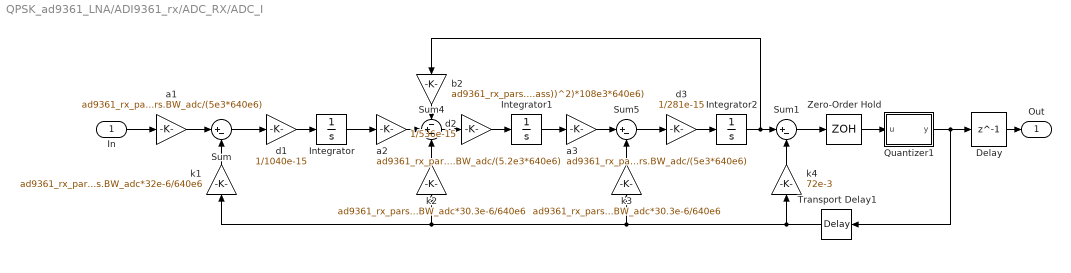
== system QPSK_ad9361_LNA/ADI9361_rx/ADC_RX/ADC_I ==
  In : Inport
  Delay : Delay  DelayLength=1
  Integrator : Integrator  LimitOutput=on  UpperSaturationLimit=0.9  LowerSaturationLimit=-0.9
  Integrator1 : Integrator  LimitOutput=on  UpperSaturationLimit=0.9  LowerSaturationLimit=-0.9
  Integrator2 : Integrator  LimitOutput=on  UpperSaturationLimit=0.9  LowerSaturationLimit=-0.9
  Quantizer1 : Subsystem
  Sum : Sum  Inputs=|+-
  Sum1 : Sum  Inputs=|+-
  Sum4 : Sum  Inputs=-+-
  Sum5 : Sum  Inputs=|+-
  Transport Delay1 : TransportDelay  DelayTime=ad9361_rx_pars.Tadc/2
  Zero-Order Hold : ZeroOrderHold  SampleTime=ad9361_rx_pars.Tadc
  a1 : Gain  Gain=ad9361_rx_pars.BW_adc/(5e3*640e6)
  a2 : Gain  Gain=ad9361_rx_pars.BW_adc/(5.2e3*640e6)
  a3 : Gain  Gain=ad9361_rx_pars.BW_adc/(5e3*640e6)
  b2 : Gain  Gain=ad9361_rx_pars.BW_adc*1024/(4*((ad9361_rx_pars.BW_adc/(2*ad9361_rx_pars.Fpass))^2)*108e3*640e6)
  d1 : Gain  Gain=1/1040e-15
  d2 : Gain  Gain=1/536e-15
  d3 : Gain  Gain=1/281e-15
  k1 : Gain  Gain=ad9361_rx_pars.BW_adc*32e-6/640e6
  k2 : Gain  Gain=ad9361_rx_pars.BW_adc*30.3e-6/640e6
  k3 : Gain  Gain=ad9361_rx_pars.BW_adc*30.3e-6/640e6
  k4 : Gain  Gain=72e-3
  Out : Outport
  wires:
  k1/1 -> Sum/2
  a1/1 -> Sum/1
  Sum5/1 -> d3/1
  Sum4/1 -> d2/1
  d3/1 -> Integrator2/1
  In/1 -> a1/1
  Integrator2/1 -> Sum1/1, b2/1
  d2/1 -> Integrator1/1
  Integrator1/1 -> a3/1
  d1/1 -> Integrator/1
  Integrator/1 -> a2/1
  Sum/1 -> d1/1
  Zero-Order Hold/1 -> Quantizer1/1(u)
  a2/1 -> Sum4/2
  k2/1 -> Sum4/3
  k3/1 -> Sum5/2
  b2/1 -> Sum4/1
  a3/1 -> Sum5/1
  Sum1/1 -> Zero-Order Hold/1
  k4/1 -> Sum1/2
  Quantizer1/1(y) -> Transport Delay1/1, Delay/1
  Transport Delay1/1 -> k4/1, k1/1, k2/1, k3/1
  Delay/1 -> Out/1

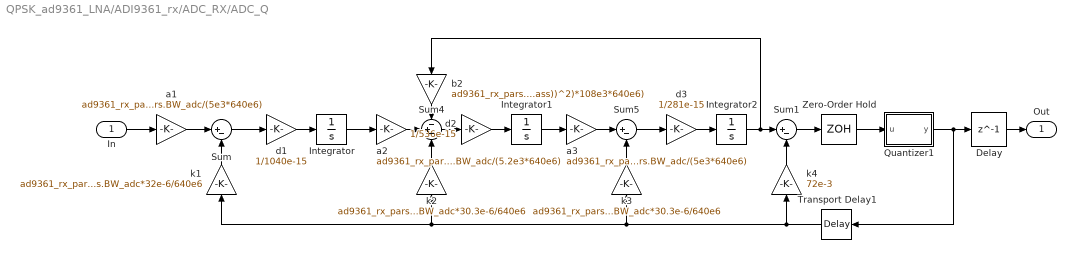
== system QPSK_ad9361_LNA/ADI9361_rx/ADC_RX/ADC_Q ==
  In : Inport
  Delay : Delay  DelayLength=1
  Integrator : Integrator  LimitOutput=on  UpperSaturationLimit=0.9  LowerSaturationLimit=-0.9
  Integrator1 : Integrator  LimitOutput=on  UpperSaturationLimit=0.9  LowerSaturationLimit=-0.9
  Integrator2 : Integrator  LimitOutput=on  UpperSaturationLimit=0.9  LowerSaturationLimit=-0.9
  Quantizer1 : Subsystem
  Sum : Sum  Inputs=|+-
  Sum1 : Sum  Inputs=|+-
  Sum4 : Sum  Inputs=-+-
  Sum5 : Sum  Inputs=|+-
  Transport Delay1 : TransportDelay  DelayTime=ad9361_rx_pars.Tadc/2
  Zero-Order Hold : ZeroOrderHold  SampleTime=ad9361_rx_pars.Tadc
  a1 : Gain  Gain=ad9361_rx_pars.BW_adc/(5e3*640e6)
  a2 : Gain  Gain=ad9361_rx_pars.BW_adc/(5.2e3*640e6)
  a3 : Gain  Gain=ad9361_rx_pars.BW_adc/(5e3*640e6)
  b2 : Gain  Gain=ad9361_rx_pars.BW_adc*1024/(4*((ad9361_rx_pars.BW_adc/(2*ad9361_rx_pars.Fpass))^2)*108e3*640e6)
  d1 : Gain  Gain=1/1040e-15
  d2 : Gain  Gain=1/536e-15
  d3 : Gain  Gain=1/281e-15
  k1 : Gain  Gain=ad9361_rx_pars.BW_adc*32e-6/640e6
  k2 : Gain  Gain=ad9361_rx_pars.BW_adc*30.3e-6/640e6
  k3 : Gain  Gain=ad9361_rx_pars.BW_adc*30.3e-6/640e6
  k4 : Gain  Gain=72e-3
  Out : Outport
  wires:
  Delay/1 -> Out/1
  Transport Delay1/1 -> k3/1, k2/1, k1/1, k4/1
  Quantizer1/1(y) -> Transport Delay1/1, Delay/1
  k4/1 -> Sum1/2
  Sum1/1 -> Zero-Order Hold/1
  a3/1 -> Sum5/1
  b2/1 -> Sum4/1
  k3/1 -> Sum5/2
  k2/1 -> Sum4/3
  a2/1 -> Sum4/2
  Zero-Order Hold/1 -> Quantizer1/1(u)
  Sum/1 -> d1/1
  Integrator/1 -> a2/1
  d1/1 -> Integrator/1
  Integrator1/1 -> a3/1
  d2/1 -> Integrator1/1
  Integrator2/1 -> b2/1, Sum1/1
  In/1 -> a1/1
  d3/1 -> Integrator2/1
  Sum4/1 -> d2/1
  Sum5/1 -> d3/1
  a1/1 -> Sum/1
  k1/1 -> Sum/2

== system QPSK_ad9361_LNA/ADI9361_rx/Average Power Meter/Peak Detector ==
  In : Inport
  HTh_i : Constant  Value=Hthreshold_i  SampleTime=ad9361_rx_pars.Tpow*Ncycles
  HTh_o : Constant  Value=Hthreshold_o  SampleTime=ad9361_rx_pars.Tpow*Ncycles
  HighThreshold : RelationalOperator  OutDataTypeStr=boolean  RndMeth=Nearest
  HighThreshold1 : RelationalOperator  Operator=<=  OutDataTypeStr=boolean  RndMeth=Nearest
  LTh_i : Constant  Value=Lthreshold_i  SampleTime=ad9361_rx_pars.Tpow*Ncycles
  LTh_o : Constant  Value=Lthreshold_o  SampleTime=ad9361_rx_pars.Tpow*Ncycles
  LowThreshold : RelationalOperator  OutDataTypeStr=boolean  RndMeth=Nearest
  LowThreshold1 : RelationalOperator  Operator=<=  OutDataTypeStr=boolean  RndMeth=Nearest
  Outer_HTh : Outport
  Inner_HTh : Outport  Port=2
  Inner_LTh : Outport  Port=3
  Outer_LTh : Outport  Port=4
  wires:
  LowThreshold/1 -> Inner_HTh/1
  HighThreshold/1 -> Outer_HTh/1
  HTh_i/1 -> LowThreshold/2
  HTh_o/1 -> HighThreshold/2
  LTh_o/1 -> LowThreshold1/2
  In/1 -> HighThreshold/1, LowThreshold1/1, HighThreshold1/1, LowThreshold/1
  LTh_i/1 -> HighThreshold1/2
  HighThreshold1/1 -> Inner_LTh/1
  LowThreshold1/1 -> Outer_LTh/1

== system QPSK_ad9361_LNA/ADI9361_rx/Average Power Meter/RMS ==
  In : Inport
  CountNCycles : Buffer  N=Ncycles
  Frame Conversion : FrameConversion  InheritSamplingMode=off  OutFrame=Sample-based
  Gain2 : Gain  Gain=1/Ncycles
  Root : Sqrt  SaturateOnIntegerOverflow=on
  Squared : Math  Operator=magnitude^2  SaturateOnIntegerOverflow=on
  Sum : Sum  Inputs=+
  Out : Outport
  wires:
  Sum/1 -> Gain2/1
  Frame Conversion/1 -> Out/1
  CountNCycles/1 -> Squared/1
  Squared/1 -> Sum/1
  Root/1 -> Frame Conversion/1
  Gain2/1 -> Root/1
  In/1 -> CountNCycles/1

== system QPSK_ad9361_LNA/ADI9361_rx/Average Power Meter/dB Conversion ==
  in : Inport
  Constant : Constant  Value=fuzz_val  OutDataTypeStr=Inherit: Inherit via back propagation  SampleTime=ad9361_rx_pars.Tpow*Ncycles
  Constant1 : Constant  Value=dBval  OutDataTypeStr=Inherit: Inherit via back propagation  SampleTime=ad9361_rx_pars.Tpow*Ncycles
  Err if non-flt : dspsigattribs/Check Signal Attributes  SigAttribCheckMethod=Does not match attributes exactly  Complexity=Ignore  Frame=Ignore  DimsCheckMethod=Ignore  Dimensions=1-D  DatatypeCheckMethod=Is...  DatatypeGeneral=Floating-point  DtypeFloatSpecific=Any floating-point  DtypeFixedSpecific=Any fixed-point  DtypeIntSpecific=Any integer  SampleMode=Ignore
      settings: SourceProductName=DSP System Toolbox  SourceProductBaseCode=DS
  Error if Cplx : dspsigattribs/Check Signal Attributes  SigAttribCheckMethod=Matches attributes exactly  Complexity=Complex  Frame=Ignore  DimsCheckMethod=Ignore  Dimensions=1-D  DatatypeCheckMethod=Ignore  DatatypeGeneral=Boolean  DtypeFloatSpecific=Any floating-point  DtypeFixedSpecific=Any fixed-point  DtypeIntSpecific=Any integer  SampleMode=Ignore
      settings: SourceProductName=DSP System Toolbox  SourceProductBaseCode=DS
  Gain : Gain  Gain=10  SaturateOnIntegerOverflow=on  OutDataTypeStr=Inherit: Same as input  ParamDataTypeStr=Inherit: Same as input
  Magsq : Math  Operator=magnitude^2  SaturateOnIntegerOverflow=on
  Scale by R : Gain  Gain=1./R  SaturateOnIntegerOverflow=on  OutDataTypeStr=Inherit: Same as input  ParamDataTypeStr=Inherit: Same as input
  Sum1 : Sum  SaturateOnIntegerOverflow=on  InputSameDT=on  OutDataTypeStr=Inherit: Same as first input
  Sum2 : Sum  SaturateOnIntegerOverflow=on  InputSameDT=on  OutDataTypeStr=Inherit: Same as first input
  log10 : Math  Operator=log10  SaturateOnIntegerOverflow=on
  out : Outport  InitialOutput=0
  wires:
  log10/1 -> Gain/1
  Magsq/1 -> Scale by R/1
  Scale by R/1 -> log10/1
  Err if non-flt/1 -> Error if Cplx/1
  in/1 -> Err if non-flt/1
  Error if Cplx/1 -> Sum1/1
  Sum1/1 -> Magsq/1
  Constant/1 -> Sum1/2
  Gain/1 -> Sum2/1
  Sum2/1 -> out/1
  Constant1/1 -> Sum2/2

== system QPSK_ad9361_LNA/ADI9361_rx/DDC_Filters_RX/Hm1 ==
  note: 1) Only subsystems can be added as variant choices at this level
      | 2) Blocks cannot be connected at this level as connectivity is
      | automatically determined at simulation, based on the active variant
  In : Inport
  Hm1 : Subsystem  VariantControl=(default)
  NoFilter : Subsystem  VariantControl=ad9361_rx_hm1Filt==0
  Out : Outport

== system QPSK_ad9361_LNA/ADI9361_rx/DDC_Filters_RX/Hm2 ==
  note: 1) Only subsystems can be added as variant choices at this level
      | 2) Blocks cannot be connected at this level as connectivity is
      | automatically determined at simulation, based on the active variant
  In : Inport
  Hm2 : Subsystem  VariantControl=(default)
  NoFilter : Subsystem  VariantControl=ad9361_rx_hm2Filt==0
  Out : Outport
